simulink model "Project_Simulation_LQR_QuestionD"  (R2018b)
settings: Solver=VariableStepAuto  StartTime=0.0  StopTime=100.0  RelTol=1e-3
values from neighbouring files (symbols this model uses):
  K = lqr(A,B,Q,R)    [PartD1.m]
settings Model: Creator=Envy  LastModifiedBy=Envy

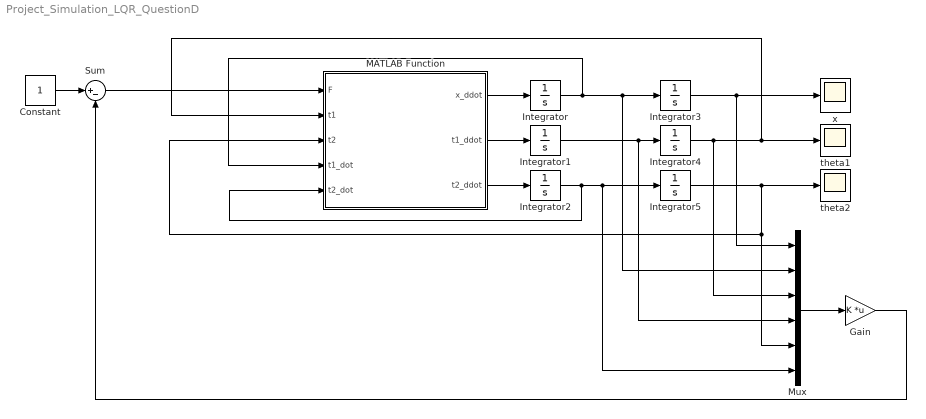
== system Project_Simulation_LQR_QuestionD ==
  Constant : Constant
  Gain : Gain  Gain=K  Multiplication=Matrix(K*u)
  Integrator{,1..5} (6 alike) : Integrator
  MATLAB Function : MATLAB Function  TreatAsAtomicUnit=on
  Mux : Mux  Inputs=6
  Sum : Sum  Inputs=|+-
  theta1 : Scope
  theta2 : Scope
  x : Scope
  wires:
  Integrator/1 -> MATLAB Function/4(t1_dot), Mux/2, Integrator3/1
  Mux/1 -> Gain/1
  Sum/1 -> MATLAB Function/1(F)
  Constant/1 -> Sum/1
  Integrator2/1 -> MATLAB Function/5(t2_dot), Mux/6, Integrator5/1
  Integrator4/1 -> Mux/3, MATLAB Function/2(t1), theta1/1
  MATLAB Function/2(t1_ddot) -> Integrator1/1
  MATLAB Function/1(x_ddot) -> Integrator/1
  Integrator1/1 -> Mux/4, Integrator4/1
  Integrator3/1 -> Mux/1, x/1
  Gain/1 -> Sum/2
  MATLAB Function/3(t2_ddot) -> Integrator2/1
  Integrator5/1 -> Mux/5, MATLAB Function/3(t2), theta2/1

== matlab function Project_Simulation_LQR_QuestionD/MATLAB Function ==
  data: F input; t1 input; t2 input; x_ddot output; t1_dot input; t2_dot input; t1_ddot output; t2_ddot output
function [x_ddot,t1_ddot,t2_ddot] = NonLinear_Simulationlqr(F,t1,t2,t1_dot,t2_dot)

%% System Parameters
l1 = 20; % length l1
l2 = 10; % length l2
m1 = 100; % mass m1
m2 = 100; % mass m2
M = 1000; % mass M
g = 9.8; % acceleration due to gravity

%% Trignometric Variables
c1 = cos(t1);
c2 = cos(t2);
s1 = sin(t1);
s2 = sin(t2);

%% x_ddot equation 
x_ddot = (F - m1*c1*s1*g - m2*c2*s2*g - m1*l1*(t1_dot^2)*(s1) - m2*l2*(t2_dot^2)*(s2))/(M + m1*(s1^2) + m2*(s2^2));

%% t1_ddot equation
t1_ddot = (x_ddot*c1 - g*s1)/l1;

%% t2_ddot equation
t2_ddot = (x_ddot*c2 - g*s2)/l2;

end
